simulink model "SIM_voltage_measurement_example"  (R2020b)
settings: Solver=VariableStepAuto  StartTime=0.0  StopTime=10.0  RelTol=1e-3
undefined symbols (not defined in the file or in its folder): Angle, Magnitude
libraries: powerlib x23
settings Model: Creator=janluca  LastModifiedBy=janluca

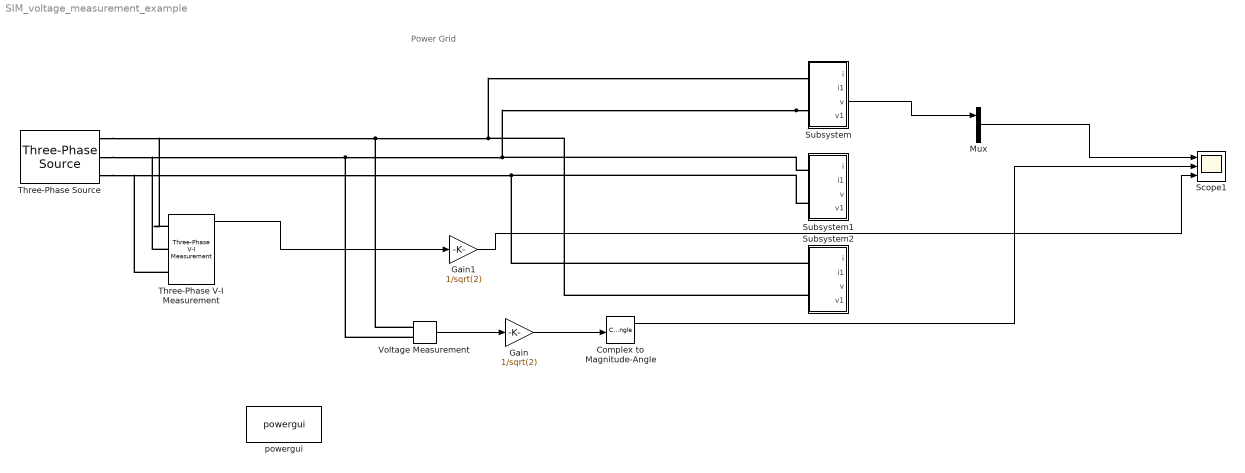
== system SIM_voltage_measurement_example ==
  note: Power Grid
  Complex to Magnitude-Angle : ComplexToMagnitudeAngle
  Gain : Gain  Gain=1/sqrt(2)
  Gain1 : Gain  Gain=1/sqrt(2)
  Mux : Mux  Inputs=3
  Scope1 : Scope  NumInputPorts=3
  Subsystem : Subsystem
  Subsystem1 : Subsystem
  Subsystem2 : Subsystem
  Three-Phase Source : powerlib/Electrical Sources/Three-Phase Source  InternalConnection=Yg  VoltagePhases=off  Voltage=230  PhaseAngle=0  Voltage_phases=[25e3 25e3 25e3]/sqrt(3)  PhaseAngles_phases=[0 -120 +120]  Frequency=50  NonIdealSource=off  SpecifyImpedance=off  Resistance=0.8929  Inductance=16.58e-3  ShortCircuitLevel=100e6  BaseVoltage=25e3  XRratio=7  BusType=PV  Pref=100  Qref=0  Prefabc=[10e3, 10e3, 10e3]  Qrefabc=[0, 0, 0]  Qmin=-inf  Qmax=inf
  Three-Phase V-I Measurement : powerlib/Measurements/Three-Phase V-I Measurement  VoltageMeasurement=phase-to-phase  SetLabelV=off  LabelV=Vabc  Vpu=off  VpuLL=off  CurrentMeasurement=no  SetLabelI=off  LabelI=Iabc  Ipu=off  Pbase=100e6  Vbase=400  OutputType=Complex  PhasorSimulation=on  PSBequivalent=0
  Voltage Measurement : powerlib/Measurements/Voltage Measurement  PhasorSimulation=on  OutputType=Complex  PSBequivalent=0
  powergui : powerlib/powergui  Priority=1  SimulationMode=Phasor  SampleTime=50e-6  frequency=50  Iterations=50  frequencyindice=50  Pbase=100e6  ErrMax=1e-4  UnitsV=kV  UnitsW=MW  buscounter=0  FunctionMessages=off  echomessages=off  EnableUseOfTLC=off  CurrentSourceSwitches=off  DisableSnubberDevices=off  DisableRonSwitches=off  DisableVfSwitches=off  DisplayEquations=off  AutomaticDiscreteSolvers=off  SolverType=Tustin/Backward Euler (TBE)  Interpol=off  ExternalGateDelay=off  methode=off  Ts=100  x0status=blocks  SPID=on  SwTol=0  HookPort=off  NonlinearTolerance=1e-4  nMaxIteration=100  ContinueOnMaxIteration=off  RestoreLinks=warning  ResistiveCurrentMeasurement=off  Frange=[0:2:500]  Ylog=off  Xlog=on  ShowGrid=off  save=off  variable=ZData  structure=0  ZoomFFT=off  StartTime=0.0  cycles=1  DisplayStyle=1  fundamental=60  FreqAxis=off  MaxFrequency=1000  frequencyindicesteady=1  RmsSteady=1  display=off
  wires:
  Mux/1 -> Scope1/1
  Voltage Measurement/1 -> Gain/1
  Three-Phase V-I Measurement/1 -> Gain1/1
  Gain1/1 -> Scope1/3
  Gain/1 -> Complex to Magnitude-Angle/1
  Complex to Magnitude-Angle/1 -> Scope1/2
  Subsystem/3(v) -> Mux/1
  connections:
  Subsystem1/LConn2 -- Three-Phase V-I Measurement/LConn3 -- Three-Phase Source/RConn3 -- Subsystem2/LConn1
  Subsystem/LConn2 -- Three-Phase V-I Measurement/LConn2 -- Three-Phase Source/RConn2 -- Voltage Measurement/LConn2 -- Subsystem1/LConn1
  Subsystem2/LConn2 -- Three-Phase V-I Measurement/LConn1 -- Three-Phase Source/RConn1 -- Voltage Measurement/LConn1 -- Subsystem/LConn1

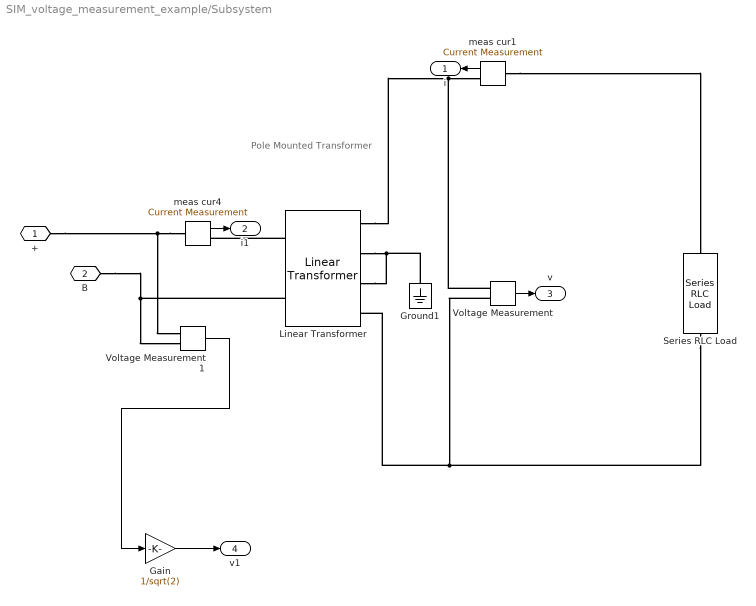
== system SIM_voltage_measurement_example/Subsystem ==
  note: Pole Mounted
      | Transformer
  Gain : Gain  Gain=1/sqrt(2)
  Ground1 : powerlib/Elements/Ground  LConnTagsString=a
  Linear Transformer : powerlib/Elements/Linear Transformer  UNITS=pu  NominalPower=[75e3 50]  winding1=[ 6600 0.00005 0.0002 ]  winding2=[ 100 0.00005 0.0002 ]  ThreeWindings=on  winding3=[ 100 0.00005 0.0002 ]  RmLm=[ 50 50 ]  Measurements=None  DataType=off
  Series RLC Load : powerlib/Elements/Series RLC Load  LConnTagsString=a  RConnTagsString=__new0  NominalVoltage=200  NominalFrequency=1  ActivePower=300  InductivePower=0  CapacitivePower=0  Setx0=off  InitialVoltage=0  SetiL0=off  InitialCurrent=0  Measurements=None  LoadType=constant PQ
  Voltage Measurement : powerlib/Measurements/Voltage Measurement  PhasorSimulation=on  OutputType=Complex  PSBequivalent=0
  Voltage Measurement1 : powerlib/Measurements/Voltage Measurement  PhasorSimulation=on  OutputType=Complex  PSBequivalent=0
  meas cur1 : powerlib/Measurements/Current Measurement  PhasorSimulation=on  OutputType=Complex  PSBequivalent=0
  meas cur4 : powerlib/Measurements/Current Measurement  PhasorSimulation=on  OutputType=Magnitude-Angle  PSBequivalent=0
  + : PMIOPort  Side=Left
  B : PMIOPort  Port=2  Side=Left
  i : Outport
  i1 : Outport  Port=2
  v : Outport  Port=3
  v1 : Outport  Port=4
  wires:
  Voltage Measurement/1 -> v/1
  meas cur1/1 -> i/1
  meas cur4/1 -> i1/1
  Gain/1 -> v1/1
  Voltage Measurement1/1 -> Gain/1
  connections:
  meas cur4/LConn1 -- Voltage Measurement1/LConn1 -- +/RConn1
  Linear Transformer/LConn2 -- Voltage Measurement1/LConn2 -- B/RConn1
  Linear Transformer/RConn1 -- meas cur1/RConn1 -- Voltage Measurement/LConn1
  Linear Transformer/LConn1 -- meas cur4/RConn1
  Linear Transformer/RConn3 -- Linear Transformer/RConn2 -- Ground1/LConn1
  Voltage Measurement/LConn2 -- Series RLC Load/RConn1 -- Linear Transformer/RConn4
  meas cur1/LConn1 -- Series RLC Load/LConn1

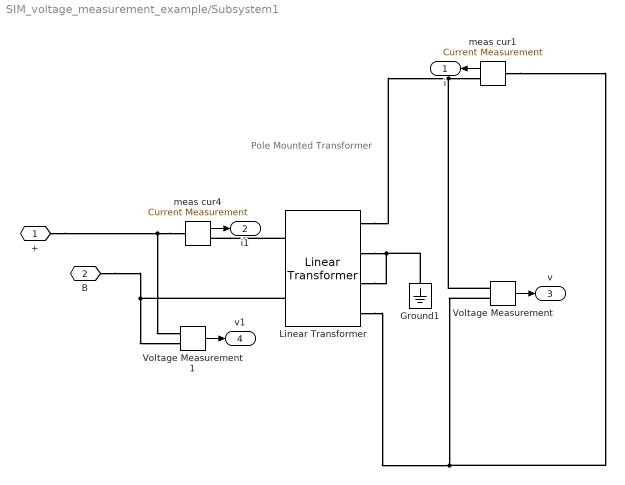
== system SIM_voltage_measurement_example/Subsystem1 ==
  note: Pole Mounted
      | Transformer
  Ground1 : powerlib/Elements/Ground  LConnTagsString=a
  Linear Transformer : powerlib/Elements/Linear Transformer  UNITS=pu  NominalPower=[75e3 50]  winding1=[ 6600 0.00005 0.0002 ]  winding2=[ 100 0.00005 0.0002 ]  ThreeWindings=on  winding3=[ 100 0.00005 0.0002 ]  RmLm=[ 50 50 ]  Measurements=None  DataType=off
  Voltage Measurement : powerlib/Measurements/Voltage Measurement  PhasorSimulation=on  OutputType=Complex  PSBequivalent=0
  Voltage Measurement1 : powerlib/Measurements/Voltage Measurement  PhasorSimulation=on  OutputType=Magnitude  PSBequivalent=0
  meas cur1 : powerlib/Measurements/Current Measurement  PhasorSimulation=on  OutputType=Complex  PSBequivalent=0
  meas cur4 : powerlib/Measurements/Current Measurement  PhasorSimulation=on  OutputType=Magnitude-Angle  PSBequivalent=0
  + : PMIOPort  Side=Left
  B : PMIOPort  Port=2  Side=Left
  i : Outport
  i1 : Outport  Port=2
  v : Outport  Port=3
  v1 : Outport  Port=4
  wires:
  Voltage Measurement/1 -> v/1
  Voltage Measurement1/1 -> v1/1
  meas cur1/1 -> i/1
  meas cur4/1 -> i1/1
  connections:
  meas cur4/LConn1 -- Voltage Measurement1/LConn1 -- +/RConn1
  Linear Transformer/LConn2 -- Voltage Measurement1/LConn2 -- B/RConn1
  Linear Transformer/RConn1 -- meas cur1/RConn1 -- Voltage Measurement/LConn1
  Linear Transformer/LConn1 -- meas cur4/RConn1
  Linear Transformer/RConn3 -- Linear Transformer/RConn2 -- Ground1/LConn1
  meas cur1/LConn1 -- Linear Transformer/RConn4 -- Voltage Measurement/LConn2

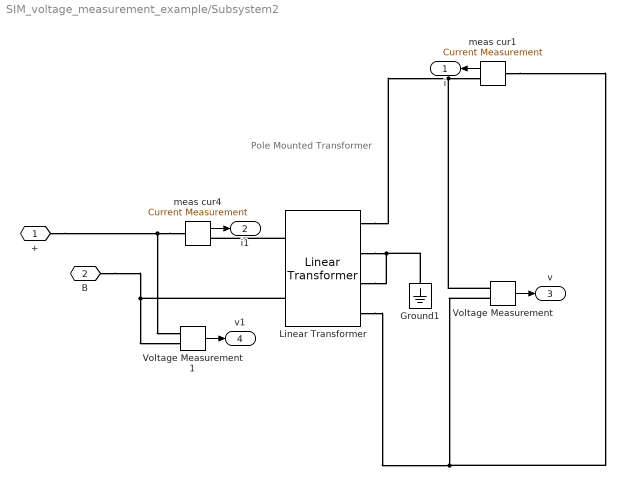
== system SIM_voltage_measurement_example/Subsystem2 ==
  note: Pole Mounted
      | Transformer
  Ground1 : powerlib/Elements/Ground  LConnTagsString=a
  Linear Transformer : powerlib/Elements/Linear Transformer  UNITS=pu  NominalPower=[75e3 50]  winding1=[ 6600 0.00005 0.0002 ]  winding2=[ 100 0.00005 0.0002 ]  ThreeWindings=on  winding3=[ 100 0.00005 0.0002 ]  RmLm=[ 50 50 ]  Measurements=None  DataType=off
  Voltage Measurement : powerlib/Measurements/Voltage Measurement  PhasorSimulation=on  OutputType=Complex  PSBequivalent=0
  Voltage Measurement1 : powerlib/Measurements/Voltage Measurement  PhasorSimulation=on  OutputType=Magnitude  PSBequivalent=0
  meas cur1 : powerlib/Measurements/Current Measurement  PhasorSimulation=on  OutputType=Complex  PSBequivalent=0
  meas cur4 : powerlib/Measurements/Current Measurement  PhasorSimulation=on  OutputType=Magnitude-Angle  PSBequivalent=0
  + : PMIOPort  Side=Left
  B : PMIOPort  Port=2  Side=Left
  i : Outport
  i1 : Outport  Port=2
  v : Outport  Port=3
  v1 : Outport  Port=4
  wires:
  Voltage Measurement/1 -> v/1
  Voltage Measurement1/1 -> v1/1
  meas cur1/1 -> i/1
  meas cur4/1 -> i1/1
  connections:
  meas cur4/LConn1 -- Voltage Measurement1/LConn1 -- +/RConn1
  Linear Transformer/LConn2 -- Voltage Measurement1/LConn2 -- B/RConn1
  Linear Transformer/RConn1 -- meas cur1/RConn1 -- Voltage Measurement/LConn1
  Linear Transformer/LConn1 -- meas cur4/RConn1
  Linear Transformer/RConn3 -- Linear Transformer/RConn2 -- Ground1/LConn1
  meas cur1/LConn1 -- Linear Transformer/RConn4 -- Voltage Measurement/LConn2
